simulink model "SASLong"  (R2020a)
settings: Solver=VariableStepAuto  StartTime=0.0  StopTime=300  RelTol=1e-3
values from neighbouring files (symbols this model uses):
  G_a_deltae_den = cell2mat(G_a_deltae_den)    [SimulinkTest.m]
  G_a_deltae_num = cell2mat(G_a_deltae_num)    [SimulinkTest.m]
  Gp_q_deltae_den = cell2mat(Gp_q_deltae_den)    [SimulinkTest.m]
  Gp_q_deltae_num = cell2mat(Gp_q_deltae_num)    [SimulinkTest.m]
  Gp_theta_deltae_den = cell2mat(Gp_theta_deltae_den)    [SimulinkTest.m]
  Gp_theta_deltae_num = cell2mat(Gp_theta_deltae_num)    [SimulinkTest.m]
  Gp_u_deltae_den = cell2mat(Gp_u_deltae_den)    [SimulinkTest.m]
  Gp_u_deltae_num = cell2mat(Gp_u_deltae_num)    [SimulinkTest.m]
  Gs_alpha_den = cell2mat(Gs_alpha_den)    [SimulinkTest.m]
  Gs_alpha_num = cell2mat(Gs_alpha_num)    [SimulinkTest.m]
  Gs_q_den = cell2mat(Gs_q_den)    [SimulinkTest.m]
  Gs_q_num = cell2mat(Gs_q_num)    [SimulinkTest.m]
  K_deltae_alpha = -0.005    [SimulinkTest.m]
  K_deltae_q = -0.005    [SimulinkTest.m]
  K_dl = 1/plane_OL.lon.G.Gthetadeltae.K_dim    [SimulinkTest.m]    (also in Trabajo2.m = 1/plane.lon.G.Gthetadeltae.K; Trabajo2_Long.m = 1/plane_OL.lon.G.Gthetadeltae.K; Utils.m = 1/G.K)
libraries: simulink x1
settings Model: Creator=Marc Vila  LastModifiedBy=Marc Vila

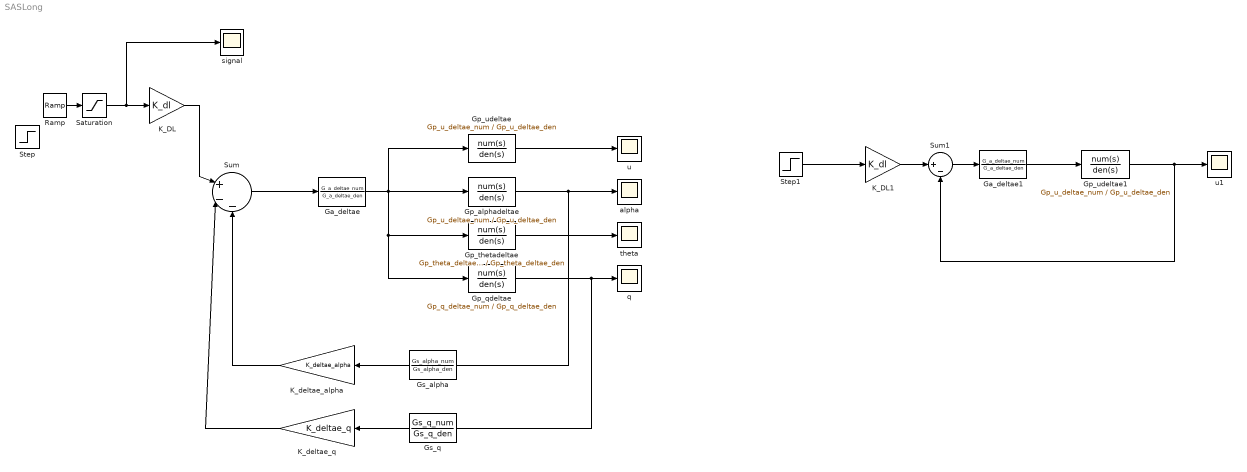
== system SASLong ==
  Ga_deltae : TransferFcn  Numerator=G_a_deltae_num  Denominator=G_a_deltae_den
  Ga_deltae1 : TransferFcn  Numerator=G_a_deltae_num  Denominator=G_a_deltae_den
  Gp_alphadeltae : TransferFcn  Numerator=Gp_u_deltae_num  Denominator=Gp_u_deltae_den
  Gp_qdeltae : TransferFcn  Numerator=Gp_q_deltae_num  Denominator=Gp_q_deltae_den
  Gp_thetadeltae : TransferFcn  Numerator=Gp_theta_deltae_num  Denominator=Gp_theta_deltae_den
  Gp_udeltae : TransferFcn  Numerator=Gp_u_deltae_num  Denominator=Gp_u_deltae_den
  Gp_udeltae1 : TransferFcn  Numerator=Gp_u_deltae_num  Denominator=Gp_u_deltae_den
  Gs_alpha : TransferFcn  Numerator=Gs_alpha_num  Denominator=Gs_alpha_den
  Gs_q : TransferFcn  Numerator=Gs_q_num  Denominator=Gs_q_den
  K_DL : Gain  Gain=K_dl
  K_DL1 : Gain  Gain=K_dl
  K_deltae_alpha : Gain  Gain=K_deltae_alpha
  K_deltae_q : Gain  Gain=K_deltae_q
  Ramp : simulink/Sources/Ramp  slope=5  start=0  InitialOutput=0
  Saturation : Saturate  UpperLimit=1  LowerLimit=0
  Step : Step  SampleTime=0
  Step1 : Step  SampleTime=0
  Sum : Sum  Inputs=|+--
  Sum1 : Sum  Inputs=|+-
  alpha : Scope
  q : Scope
  signal : Scope
      settings: Tag=u
  theta : Scope
  u : Scope
      settings: Tag=u
  u1 : Scope
      settings: Tag=u
  wires:
  Gp_qdeltae/1 -> K_deltae_q/1, q/1
  Gp_thetadeltae/1 -> theta/1
  Gp_alphadeltae/1 -> K_deltae_alpha/1, alpha/1
  Gp_udeltae/1 -> u/1
  K_DL/1 -> Sum/1
  K_deltae_alpha/1 -> Sum/3
  K_deltae_q/1 -> Sum/2
  Sum/1 -> Ga_deltae/1
  Ga_deltae/1 -> Gp_qdeltae/1, Gp_thetadeltae/1, Gp_udeltae/1, Gp_alphadeltae/1
  Ga_deltae1/1 -> Gp_udeltae1/1
  Step1/1 -> K_DL1/1
  K_DL1/1 -> Sum1/1
  Sum1/1 -> Ga_deltae1/1
  Gp_udeltae1/1 -> Sum1/2, u1/1
  Ramp/1 -> Saturation/1
  Saturation/1 -> signal/1, K_DL/1
